simulink model "gaintable_sim"  (R2020b)
settings: Solver=FixedStepAuto  StartTime=0.0  StopTime=stop_time  RelTol=1e-3
InitFcn:
  | gaintable_sim_init
StopFcn:
  | gaintable_sim_stop
values from neighbouring files (symbols this model uses):
  band_number = 1:num_bands    [gaintable_sim_init.m]
  fs = 48e3    (= 48000)    [gaintable_sim_init.m]
  num_bands = 8    [gaintable_sim_init.m]
settings Model: Creator=t96f346  LastModifiedBy=wickh
settings DataIOCC: ReturnWorkspaceOutputs=off
settings OptimizationCC: BlockReduction=off  ConditionallyExecuteInputs=off  DefaultParameterBehavior=Inlined
settings DebuggingCC: AlgebraicLoopMsg=error
settings HardwareCC: ProdBitPerPointer=32  ProdBitPerSizeT=32  ProdBitPerPtrDiffT=32  ProdLargestAtomicFloat=None  ProdIntDivRoundTo=Undefined  ProdEndianess=Unspecified  ProdWordSize=32  ProdHWDeviceType=ASIC/FPGA->ASIC/FPGA  TargetBitPerPointer=64  TargetBitPerSizeT=64  TargetBitPerPtrDiffT=64  TargetLongLongMode=on  TargetIntDivRoundTo=Zero  TargetEndianess=LittleEndian  TargetWordSize=64  TargetHWDeviceType=Custom Processor->MATLAB Host Computer  ProdEqTarget=off

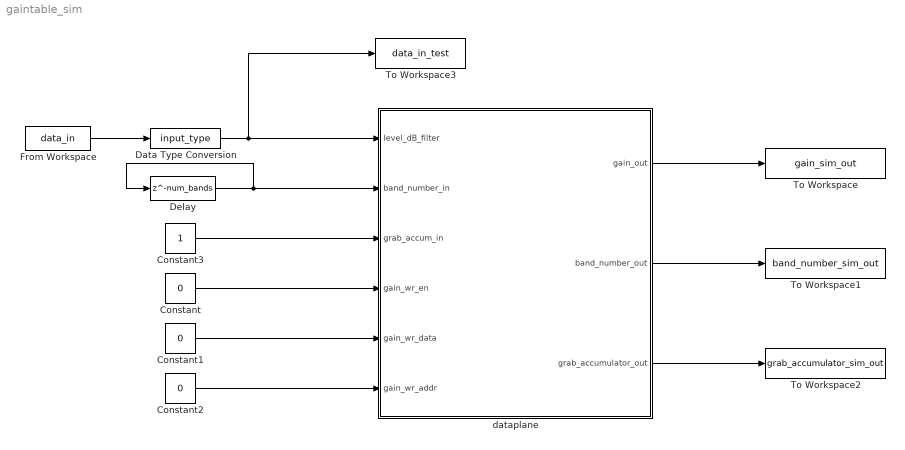
== system gaintable_sim ==
  Constant : Constant  Value=0  OutDataTypeStr=boolean  SampleTime=-1
  Constant1 : Constant  Value=0  OutDataTypeStr=gain_coeff_type  SampleTime=-1
  Constant2 : Constant  Value=0  OutDataTypeStr=uint8  SampleTime=-1
  Constant3 : Constant  OutDataTypeStr=boolean  SampleTime=-1
  Data Type Conversion : DataTypeConversion  OutDataTypeStr=input_type
  Delay : Delay  DelayLength=num_bands  InitialCondition=band_number
  From Workspace : FromWorkspace  VariableName=data_in  SampleTime=1/fs  Interpolate=off  OutputAfterFinalValue=Holding final value
  To Workspace : ToWorkspace  VariableName=gain_sim_out  SampleTime=-1
  To Workspace1 : ToWorkspace  VariableName=band_number_sim_out  SampleTime=-1
  To Workspace2 : ToWorkspace  VariableName=grab_accumulator_sim_out  SampleTime=-1
  To Workspace3 : ToWorkspace  VariableName=data_in_test  SampleTime=-1
  dataplane : Subsystem
  wires:
  Delay/1 -> Delay/1, dataplane/2(band_number_in)
  From Workspace/1 -> Data Type Conversion/1
  Data Type Conversion/1 -> To Workspace3/1, dataplane/1(level_dB_filter)
  Constant3/1 -> dataplane/3(grab_accum_in)
  Constant/1 -> dataplane/4(gain_wr_en)
  Constant1/1 -> dataplane/5(gain_wr_data)
  Constant2/1 -> dataplane/6(gain_wr_addr)
  dataplane/3(grab_accumulator_out) -> To Workspace2/1
  dataplane/2(band_number_out) -> To Workspace1/1
  dataplane/1(gain_out) -> To Workspace/1

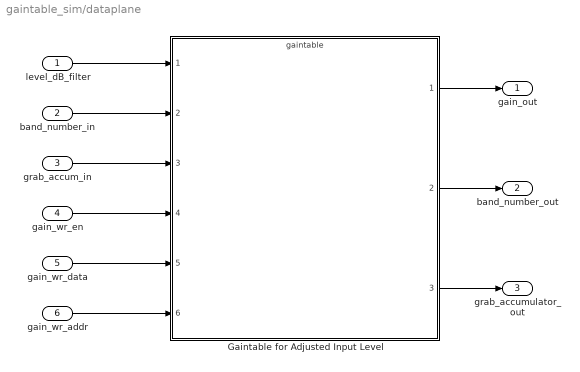
== system gaintable_sim/dataplane ==
  level_dB_filter : Inport
  band_number_in : Inport  Port=2
  grab_accum_in : Inport  Port=3
  gain_wr_en : Inport  Port=4
  gain_wr_data : Inport  Port=5
  gain_wr_addr : Inport  Port=6
  Gaintable for Adjusted Input Level : ModelReference  ModelNameDialog=gaintable  SimulationMode=Normal  ModelReferenceVersion=2.75
  gain_out : Outport
  band_number_out : Outport  Port=2
  grab_accumulator_out : Outport  Port=3
  wires:
  Gaintable for Adjusted Input Level/1 -> gain_out/1
  Gaintable for Adjusted Input Level/2 -> band_number_out/1
  Gaintable for Adjusted Input Level/3 -> grab_accumulator_out/1
  level_dB_filter/1 -> Gaintable for Adjusted Input Level/1
  band_number_in/1 -> Gaintable for Adjusted Input Level/2
  grab_accum_in/1 -> Gaintable for Adjusted Input Level/3
  gain_wr_en/1 -> Gaintable for Adjusted Input Level/4
  gain_wr_data/1 -> Gaintable for Adjusted Input Level/5
  gain_wr_addr/1 -> Gaintable for Adjusted Input Level/6
